simulink model "getDataSim"  (R2013a)
settings: Solver=ode45  StartTime=0.0  StopTime=t  RelTol=1e-3
values from neighbouring files (symbols this model uses):
  sampleTime = mydata.sampleTime    [runtracklsq.m]    (also in workspace.mat = 0.01)
undefined symbols (not defined in the file or in its folder): sampleTimeCam
libraries: aerolibutil x1
settings Model: Creator=User  LastModifiedBy=User

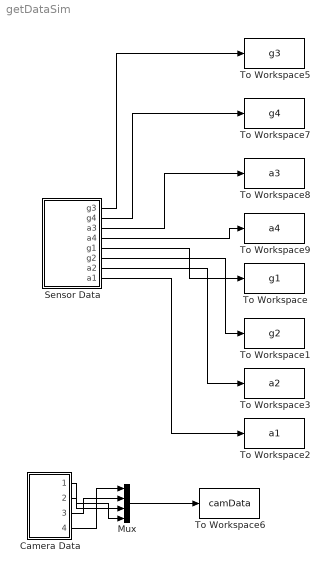
== system getDataSim ==
  Camera Data : Subsystem
  Mux : Mux
  Sensor Data : Subsystem
  To Workspace : ToWorkspace  VariableName=g1  SampleTime=sampleTime  SaveFormat=Structure With Time
  To Workspace1 : ToWorkspace  VariableName=g2  SampleTime=sampleTime  SaveFormat=Structure With Time
  To Workspace2 : ToWorkspace  VariableName=a1  SampleTime=sampleTime  SaveFormat=Structure With Time
  To Workspace3 : ToWorkspace  VariableName=a2  SampleTime=sampleTime  SaveFormat=Structure With Time
  To Workspace5 : ToWorkspace  VariableName=g3  SampleTime=sampleTime  SaveFormat=Structure With Time
  To Workspace6 : ToWorkspace  VariableName=camData  SampleTime=sampleTime  SaveFormat=Structure With Time
  To Workspace7 : ToWorkspace  VariableName=g4  SampleTime=sampleTime  SaveFormat=Structure With Time
  To Workspace8 : ToWorkspace  VariableName=a3  SampleTime=sampleTime  SaveFormat=Structure With Time
  To Workspace9 : ToWorkspace  VariableName=a4  SampleTime=sampleTime  SaveFormat=Structure With Time
  wires:
  Mux/1 -> To Workspace6/1
  Sensor Data/8(a1) -> To Workspace2/1
  Sensor Data/7(a2) -> To Workspace3/1
  Sensor Data/6(g2) -> To Workspace1/1
  Sensor Data/5(g1) -> To Workspace/1
  Sensor Data/4(a4) -> To Workspace9/1
  Sensor Data/3(a3) -> To Workspace8/1
  Sensor Data/2("g4 ") -> To Workspace7/1
  Sensor Data/1("g3 ") -> To Workspace5/1
  Camera Data/4(camS1) -> Mux/1
  Camera Data/3(cams2) -> Mux/2
  Camera Data/1(cams3) -> Mux/3
  Camera Data/2(cams4) -> Mux/4

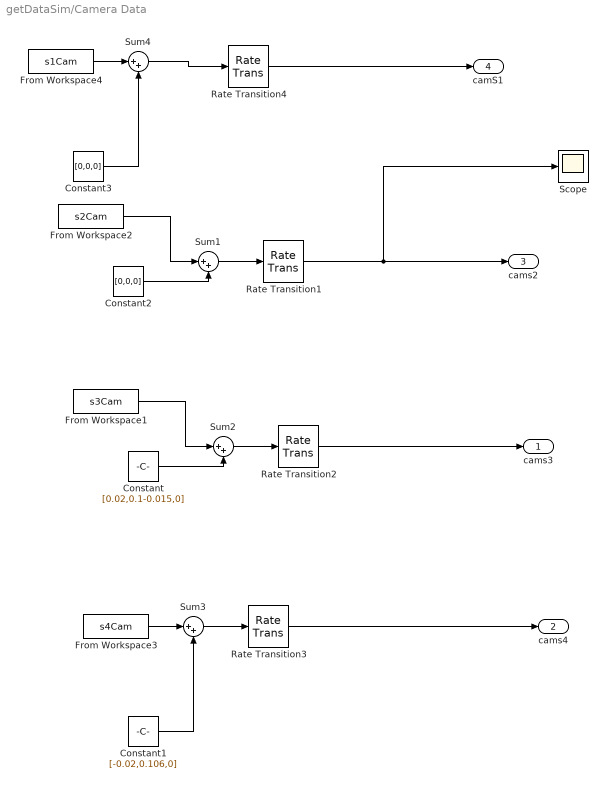
== system getDataSim/Camera Data ==
  Constant : Constant  Value=[0.02,0.1-0.015,0]
  Constant1 : Constant  Value=[-0.02,0.106,0]
  Constant2 : Constant  Value=[0,0,0]
  Constant3 : Constant  Value=[0,0,0]
  From Workspace1 : FromWorkspace  VariableName=s3Cam  SampleTime=sampleTimeCam
  From Workspace2 : FromWorkspace  VariableName=s2Cam  SampleTime=sampleTimeCam
  From Workspace3 : FromWorkspace  VariableName=s4Cam  SampleTime=sampleTimeCam
  From Workspace4 : FromWorkspace  VariableName=s1Cam  SampleTime=sampleTimeCam
  Rate Transition{1..4} (4 alike) : RateTransition  Deterministic=off
  Scope : Scope
      settings: SaveName=ScopeData12
  Sum{1..4} (4 alike) : Sum  Inputs=|++
  cams3 : Outport
  cams4 : Outport  Port=2
  cams2 : Outport  Port=3
  camS1 : Outport  Port=4
  wires:
  Sum3/1 -> Rate Transition3/1
  From Workspace1/1 -> Sum2/1
  Constant/1 -> Sum2/2
  Rate Transition2/1 -> cams3/1
  Constant1/1 -> Sum3/2
  Sum2/1 -> Rate Transition2/1
  From Workspace3/1 -> Sum3/1
  Rate Transition3/1 -> cams4/1
  From Workspace2/1 -> Sum1/1
  Constant2/1 -> Sum1/2
  Rate Transition1/1 -> Scope/1, cams2/1
  Sum1/1 -> Rate Transition1/1
  Rate Transition4/1 -> camS1/1
  Sum4/1 -> Rate Transition4/1
  Constant3/1 -> Sum4/2
  From Workspace4/1 -> Sum4/1

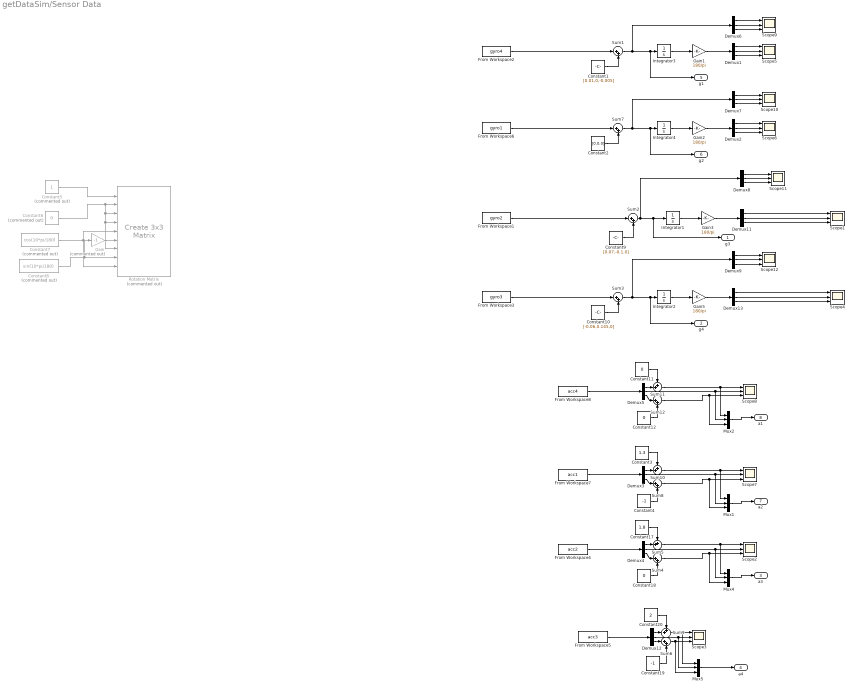
== system getDataSim/Sensor Data ==
  Constant1 : Constant  Value=[0.01,0,-0.005]
  Constant10 : Constant  Value=[-0.06,0.145,0]
  Constant11 : Constant  Value=0
  Constant12 : Constant  Value=0
  Constant17 : Constant  Value=1.8
  Constant18 : Constant  Value=0
  Constant19 : Constant  Value=-1
  Constant2 : Constant  Value=[0,0,0]
  Constant20 : Constant  Value=2
  Constant3 : Constant  Value=1.3
  Constant4 : Constant  Value=-1
  Constant5 : Constant  Commented=on
  Constant6 : Constant  Commented=on  Value=0
  Constant7 : Constant  Commented=on  Value=cos(10*pi/180)
  Constant8 : Constant  Commented=on  Value=sin(10*pi/180)
  Constant9 : Constant  Value=[0.07,-0.1,0]
  Demux{1..9,11..13} (12 alike) : Demux  Outputs=3
  From Workspace1 : FromWorkspace  VariableName=gyro2  SampleTime=sampleTime
  From Workspace2 : FromWorkspace  VariableName=gyro4  SampleTime=sampleTime
  From Workspace3 : FromWorkspace  VariableName=gyro3  SampleTime=sampleTime
  From Workspace4 : FromWorkspace  VariableName=acc2  SampleTime=sampleTime
  From Workspace5 : FromWorkspace  VariableName=acc3  SampleTime=sampleTime
  From Workspace6 : FromWorkspace  VariableName=gyro1  SampleTime=sampleTime
  From Workspace7 : FromWorkspace  VariableName=acc1  SampleTime=sampleTime
  From Workspace8 : FromWorkspace  VariableName=acc4  SampleTime=sampleTime
  Gain : Gain  Commented=on  Gain=-1
  Gain{1..3,5} (4 alike) : Gain  Gain=180/pi
  Integrator{1..4} (4 alike) : Integrator
  Mux{1..2,4..5} (4 alike) : Mux  Inputs=3
  Rotation Matrix : aerolibutil/Create 3x3 Matrix  Commented=on
  Scope{1..12} (12 alike) : Scope  NumInputPorts=3
      Scope1 settings: TimeRange=6  YMin=-35~-35~-35  YMax=0~5~5
      Scope10 settings: YMin=-5~-5~-5  YMax=5~5~5  SaveName=ScopeData9
      Scope11 settings: YMin=-5~-5~-5  YMax=5~5~5  SaveName=ScopeData10
      Scope12 settings: YMin=-5~-5~-5  YMax=5~5~5  SaveName=ScopeData11
      Scope2 settings: YMin=-5~-5~-5  YMax=5~5~5
      Scope3 settings: YMin=-5~-5~-5  YMax=5~5~5  SaveName=ScopeData2
      Scope4 settings: YMin=-5~-5~-5  YMax=5~5~5  SaveName=ScopeData3
      Scope5 settings: YMin=-5~-5~-5  YMax=5~5~5  SaveName=ScopeData4
      Scope6 settings: YMin=-5~-5~-5  YMax=5~5~5  SaveName=ScopeData5
      Scope7 settings: YMin=-5~-5~-5  YMax=5~5~5  SaveName=ScopeData6
      Scope8 settings: YMin=-5~-5~-5  YMax=5~5~5  SaveName=ScopeData7
      Scope9 settings: YMin=-5~-5~-5  YMax=5~5~5  SaveName=ScopeData8
  Sum{1..4,6..8,12} (8 alike) : Sum  Inputs=|++
  Sum{5,9..11} (4 alike) : Sum  Inputs=++|
  "g3 " : Outport
  "g4 " : Outport  Port=2
  a3 : Outport  Port=3
  a4 : Outport  Port=4
  g1 : Outport  Port=5
  g2 : Outport  Port=6
  a2 : Outport  Port=7
  a1 : Outport  Port=8
  wires:
  Constant5/1 -> Rotation Matrix/1
  Constant6/1 -> Rotation Matrix/7, Rotation Matrix/4, Rotation Matrix/3, Rotation Matrix/2
  Constant7/1 -> Rotation Matrix/5, Rotation Matrix/9
  Constant8/1 -> Gain/1, Rotation Matrix/8
  Gain/1 -> Rotation Matrix/6
  Integrator1/1 -> Gain3/1
  Demux11/1 -> Scope1/1
  Demux11/2 -> Scope1/2
  Demux11/3 -> Scope1/3
  Gain3/1 -> Demux11/1
  From Workspace1/1 -> Sum2/1
  Constant9/1 -> Sum2/2
  Demux13/1 -> Scope4/1
  Demux13/2 -> Scope4/2
  Demux13/3 -> Scope4/3
  Integrator2/1 -> Gain5/1
  Gain5/1 -> Demux13/1
  From Workspace3/1 -> Sum3/1
  Constant10/1 -> Sum3/2
  From Workspace4/1 -> Demux4/1
  Sum5/1 -> Mux4/1, Scope2/1
  Demux4/2 -> Mux4/2, Scope2/2
  Sum4/1 -> Mux4/3, Scope2/3
  Demux4/3 -> Sum4/1
  Constant18/1 -> Sum4/2
  Demux4/1 -> Sum5/2
  Constant17/1 -> Sum5/1
  Mux4/1 -> a3/1
  From Workspace5/1 -> Demux12/1
  Sum9/1 -> Mux5/1, Scope3/1
  Demux12/2 -> Mux5/2, Scope3/2
  Sum6/1 -> Mux5/3, Scope3/3
  Demux12/3 -> Sum6/1
  Constant19/1 -> Sum6/2
  Demux12/1 -> Sum9/2
  Constant20/1 -> Sum9/1
  Mux5/1 -> a4/1
  Demux1/1 -> Scope5/1
  Demux1/2 -> Scope5/2
  Demux1/3 -> Scope5/3
  Integrator3/1 -> Gain1/1
  Gain1/1 -> Demux1/1
  From Workspace2/1 -> Sum1/1
  Constant1/1 -> Sum1/2
  Demux2/1 -> Scope6/1
  Demux2/2 -> Scope6/2
  Demux2/3 -> Scope6/3
  Integrator4/1 -> Gain2/1
  Gain2/1 -> Demux2/1
  From Workspace6/1 -> Sum7/1
  Constant2/1 -> Sum7/2
  From Workspace7/1 -> Demux3/1
  Sum10/1 -> Mux1/1, Scope7/1
  Demux3/2 -> Mux1/2, Scope7/2
  Sum8/1 -> Mux1/3, Scope7/3
  Demux3/3 -> Sum8/1
  Constant4/1 -> Sum8/2
  Demux3/1 -> Sum10/2
  Constant3/1 -> Sum10/1
  Mux1/1 -> a2/1
  From Workspace8/1 -> Demux5/1
  Sum11/1 -> Mux2/1, Scope8/1
  Demux5/2 -> Mux2/2, Scope8/2
  Sum12/1 -> Mux2/3, Scope8/3
  Demux5/3 -> Sum12/1
  Constant12/1 -> Sum12/2
  Demux5/1 -> Sum11/2
  Constant11/1 -> Sum11/1
  Mux2/1 -> a1/1
  Demux6/1 -> Scope9/1
  Demux6/2 -> Scope9/2
  Demux6/3 -> Scope9/3
  Sum1/1 -> Demux6/1, g1/1, Integrator3/1
  Demux7/1 -> Scope10/1
  Demux7/2 -> Scope10/2
  Demux7/3 -> Scope10/3
  Sum7/1 -> Demux7/1, g2/1, Integrator4/1
  Demux8/1 -> Scope11/1
  Demux8/2 -> Scope11/2
  Demux8/3 -> Scope11/3
  Sum2/1 -> Demux8/1, "g3 "/1, Integrator1/1
  Demux9/1 -> Scope12/1
  Demux9/2 -> Scope12/2
  Demux9/3 -> Scope12/3
  Sum3/1 -> Demux9/1, "g4 "/1, Integrator2/1
